simulink model "lqe_model"  (R2024a)
settings: Solver=FixedStepAuto  StartTime=0.0  StopTime=10  FixedStep=0.0001  RelTol=1e-3
values from neighbouring files (symbols this model uses):
  A = [20 5 -16 9; 6 1 -4 1; 32 9 -25 14; 8 4 -6 4]    [lqe.m]    (also in lqg.m = [5 -5 -9 3; -5 5 -3 9; -9 -3 5 5; 3 9 5 5]; lqr.m = [11 -2 13; 6 -1 6; -6 -1 -8])
  C = [-1 0 1 -1]    [lqe.m]    (also in lqg.m = [1 -1 1 1; 1 3 -1 3])
  fa1 = 1/4    (= 0.25)    [lqe.m]
  fa2 = 2/4    (= 0.5)    [lqe.m]
  fa3 = 3/4    (= 0.75)    [lqe.m]
  fa4 = 4/4    (= 1)    [lqe.m]
  fw1 = 2    [lqe.m]
  fw2 = 4    [lqe.m]
  fw3 = 1    [lqe.m]
  fw4 = 3    [lqe.m]
  ksia = 1    [lqe.m]
  ksiw = 5    [lqe.m]
  L = L1    [lqe.m]    (also in lqg.m = -Pl*C'/Rl)
  L1 = -P1*C'/R1    [lqe.m]
  L2 = -P2*C'/R2    [lqe.m]
  L3 = -P3*C'/R3    [lqe.m]
  L4 = -P4*C'/R4    [lqe.m]
settings Model: Creator=ventus  LastModifiedBy=ventus

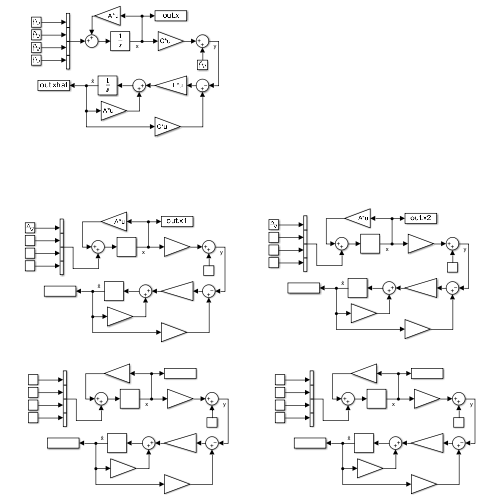
[thumbnail: Simulink's stored preview of the top-level diagram]
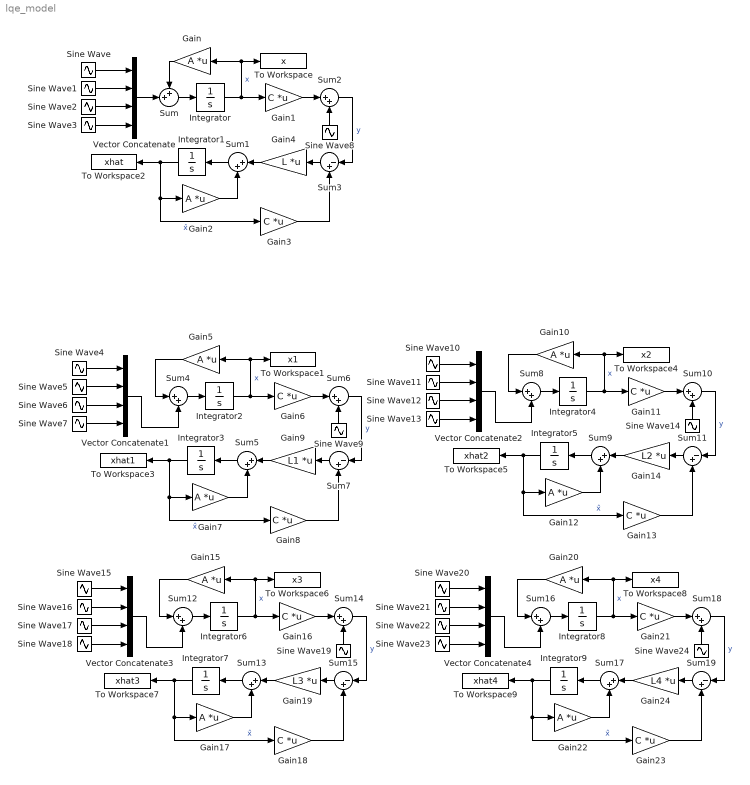
== system lqe_model ==
  Gain{,2,5,7,10,12,15,17,20,22} (10 alike) : Gain  Gain=A  Multiplication=Matrix(K*u)
  Gain{1,3,6,8,11,13,16,18,21,23} (10 alike) : Gain  Gain=C  Multiplication=Matrix(K*u)
  Gain14 : Gain  Gain=L2  Multiplication=Matrix(K*u)
  Gain19 : Gain  Gain=L3  Multiplication=Matrix(K*u)
  Gain24 : Gain  Gain=L4  Multiplication=Matrix(K*u)
  Gain4 : Gain  Gain=L  Multiplication=Matrix(K*u)
  Gain9 : Gain  Gain=L1  Multiplication=Matrix(K*u)
  Integrator{,2,4,6,8} (5 alike) : Integrator  InitialCondition=[1; 1; 1; 1]
  Integrator{1,3,5,7,9} (5 alike) : Integrator  InitialCondition=[0; 0; 0; 0]
  Sine Wave : Sin  Amplitude=fa1  Frequency=fw1  Phase=pi/2  SampleTime=0  VectorParams1D=off
  Sine Wave1 : Sin  Amplitude=fa2  Frequency=fw2  SampleTime=0  VectorParams1D=off
  Sine Wave{4,10,15,20} (4 alike) : Sin  Amplitude=fa1  Frequency=2*pi*fw1  SampleTime=0  VectorParams1D=off
  Sine Wave{5,11,16,21} (4 alike) : Sin  Amplitude=fa2  Frequency=2*pi*fw2  SampleTime=0  VectorParams1D=off
  Sine Wave{6,12,17,22} (4 alike) : Sin  Amplitude=fa3  Frequency=2*pi*fw3  Phase=pi/2  SampleTime=0  VectorParams1D=off
  Sine Wave{7,13,18,23} (4 alike) : Sin  Amplitude=fa4  Frequency=2*pi*fw4  SampleTime=0  VectorParams1D=off
  Sine Wave{9,14,19,24} (4 alike) : Sin  Amplitude=ksia  Frequency=2*pi*ksiw  SampleTime=0
  Sine Wave2 : Sin  Amplitude=fa3  Frequency=fw3  Phase=pi/2  SampleTime=0  VectorParams1D=off
  Sine Wave3 : Sin  Amplitude=fa4  Frequency=fw4  SampleTime=0  VectorParams1D=off
  Sine Wave8 : Sin  Amplitude=ksia  Frequency=ksiw  SampleTime=0
  Sum : Sum  Inputs=++|
  Sum{1..2,4..6,8..10,12..14,16..18} (14 alike) : Sum  Inputs=|++
  Sum{3,7,11,15,19} (5 alike) : Sum  Inputs=|-+
  To Workspace : ToWorkspace  VariableName=x  SaveFormat=Timeseries  SampleTime=-1
  To Workspace1 : ToWorkspace  VariableName=x1  SaveFormat=Timeseries  SampleTime=-1
  To Workspace2 : ToWorkspace  VariableName=xhat  SaveFormat=Timeseries  SampleTime=-1
  To Workspace3 : ToWorkspace  VariableName=xhat1  SaveFormat=Timeseries  SampleTime=-1
  To Workspace4 : ToWorkspace  VariableName=x2  SaveFormat=Timeseries  SampleTime=-1
  To Workspace5 : ToWorkspace  VariableName=xhat2  SaveFormat=Timeseries  SampleTime=-1
  To Workspace6 : ToWorkspace  VariableName=x3  SaveFormat=Timeseries  SampleTime=-1
  To Workspace7 : ToWorkspace  VariableName=xhat3  SaveFormat=Timeseries  SampleTime=-1
  To Workspace8 : ToWorkspace  VariableName=x4  SaveFormat=Timeseries  SampleTime=-1
  To Workspace9 : ToWorkspace  VariableName=xhat4  SaveFormat=Timeseries  SampleTime=-1
  Vector Concatenate{,1..4} (5 alike) : Concatenate  NumInputs=4
  wires:
  Integrator/1 -> Gain/1, To Workspace/1, Gain1/1  "x"
  Gain/1 -> Sum/1
  Sum/1 -> Integrator/1
  Sine Wave3/1 -> Vector Concatenate/4
  Sine Wave2/1 -> Vector Concatenate/3
  Sine Wave1/1 -> Vector Concatenate/2
  Sine Wave/1 -> Vector Concatenate/1
  Vector Concatenate/1 -> Sum/2
  Sum2/1 -> Sum3/1  "y"
  Sine Wave8/1 -> Sum2/2
  Gain1/1 -> Sum2/1
  Sum1/1 -> Integrator1/1
  Integrator1/1 -> To Workspace2/1, Gain3/1, Gain2/1  "x̂"
  Gain2/1 -> Sum1/2
  Gain4/1 -> Sum1/1
  Sum3/1 -> Gain4/1
  Gain3/1 -> Sum3/2
  Gain9/1 -> Sum5/1
  Gain8/1 -> Sum7/2
  Sum5/1 -> Integrator3/1
  Sine Wave9/1 -> Sum6/2
  Sine Wave4/1 -> Vector Concatenate1/1
  Sine Wave7/1 -> Vector Concatenate1/4
  Sine Wave5/1 -> Vector Concatenate1/2
  Vector Concatenate1/1 -> Sum4/2
  Integrator3/1 -> To Workspace3/1, Gain8/1, Gain7/1  "x̂"
  Sine Wave6/1 -> Vector Concatenate1/3
  Gain7/1 -> Sum5/2
  Sum7/1 -> Gain9/1
  Gain6/1 -> Sum6/1
  Integrator2/1 -> Gain5/1, To Workspace1/1, Gain6/1  "x"
  Sum4/1 -> Integrator2/1
  Gain5/1 -> Sum4/1
  Sum6/1 -> Sum7/1  "y"
  Gain14/1 -> Sum9/1
  Gain13/1 -> Sum11/2
  Sum9/1 -> Integrator5/1
  Sine Wave14/1 -> Sum10/2
  Sine Wave10/1 -> Vector Concatenate2/1
  Sine Wave13/1 -> Vector Concatenate2/4
  Sine Wave11/1 -> Vector Concatenate2/2
  Vector Concatenate2/1 -> Sum8/2
  Integrator5/1 -> To Workspace5/1, Gain13/1, Gain12/1  "x̂"
  Sine Wave12/1 -> Vector Concatenate2/3
  Gain12/1 -> Sum9/2
  Sum11/1 -> Gain14/1
  Gain11/1 -> Sum10/1
  Integrator4/1 -> Gain10/1, To Workspace4/1, Gain11/1  "x"
  Sum8/1 -> Integrator4/1
  Gain10/1 -> Sum8/1
  Sum10/1 -> Sum11/1  "y"
  Gain19/1 -> Sum13/1
  Gain18/1 -> Sum15/2
  Sum13/1 -> Integrator7/1
  Sine Wave19/1 -> Sum14/2
  Sine Wave15/1 -> Vector Concatenate3/1
  Sine Wave18/1 -> Vector Concatenate3/4
  Sine Wave16/1 -> Vector Concatenate3/2
  Vector Concatenate3/1 -> Sum12/2
  Integrator7/1 -> To Workspace7/1, Gain18/1, Gain17/1  "x̂"
  Sine Wave17/1 -> Vector Concatenate3/3
  Gain17/1 -> Sum13/2
  Sum15/1 -> Gain19/1
  Gain16/1 -> Sum14/1
  Integrator6/1 -> Gain15/1, To Workspace6/1, Gain16/1  "x"
  Sum12/1 -> Integrator6/1
  Gain15/1 -> Sum12/1
  Sum14/1 -> Sum15/1  "y"
  Gain24/1 -> Sum17/1
  Gain23/1 -> Sum19/2
  Sum17/1 -> Integrator9/1
  Sine Wave24/1 -> Sum18/2
  Sine Wave20/1 -> Vector Concatenate4/1
  Sine Wave23/1 -> Vector Concatenate4/4
  Sine Wave21/1 -> Vector Concatenate4/2
  Vector Concatenate4/1 -> Sum16/2
  Integrator9/1 -> To Workspace9/1, Gain23/1, Gain22/1  "x̂"
  Sine Wave22/1 -> Vector Concatenate4/3
  Gain22/1 -> Sum17/2
  Sum19/1 -> Gain24/1
  Gain21/1 -> Sum18/1
  Integrator8/1 -> Gain20/1, To Workspace8/1, Gain21/1  "x"
  Sum16/1 -> Integrator8/1
  Gain20/1 -> Sum16/1
  Sum18/1 -> Sum19/1  "y"
